simulink model "Simulink3D"  (R2013b)
settings: Solver=ode3  StartTime=0.0  StopTime=20  RelTol=1e-3
settings Model: Creator=ThiagoCordeiro  LastModifiedBy=ThiagoFelippe

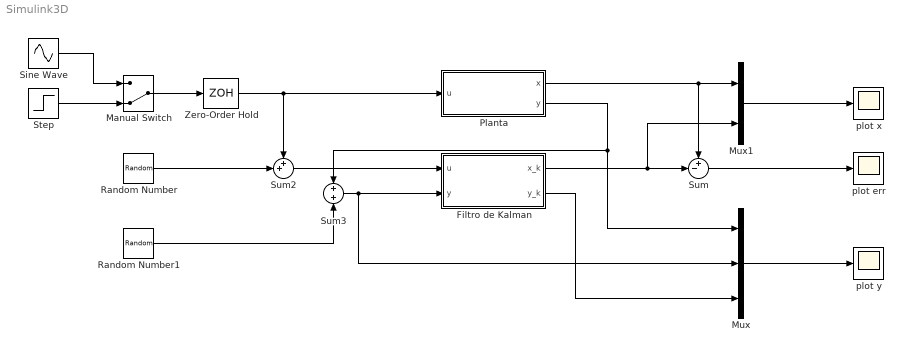
== system Simulink3D ==
  Filtro de Kalman : Subsystem
  Manual Switch : ManualSwitch  CurrentSetting=0
  Mux : Mux  Inputs=3
  Mux1 : Mux  Inputs=2
  Planta : Subsystem
  Random Number : RandomNumber  Seed=round(rand(3,1)*(2^32-1))  SampleTime=0.01
  Random Number1 : RandomNumber  Seed=round(rand(6,1)*(2^32-1))  SampleTime=0.01
  Sine Wave : Sin  Amplitude=[1 1 1]  Frequency=[1 0.5 0.25]  Phase=pi/2 * [1 1 1]  SampleTime=0
  Step : Step  Time=0  After=[2*pi/10, pi/10, pi/20]  SampleTime=0
  Sum : Sum  Inputs=+-|
  Sum2 : Sum  Inputs=++|
  Sum3 : Sum  Inputs=+|+
  Zero-Order Hold : ZeroOrderHold  SampleTime=0.01
  plot err : Scope
  plot x : Scope
  plot y : Scope
      settings: ShowLegends=on  SaveName=ScopeData2
  wires:
  Mux/1 -> plot y/1
  Zero-Order Hold/1 -> Planta/1(u), Sum2/1
  Random Number/1 -> Sum2/2
  Random Number1/1 -> Sum3/2
  Sum2/1 -> Filtro de Kalman/1(u)
  Sum3/1 -> Mux/2, Filtro de Kalman/2(y)
  Planta/2(y) -> Mux/1, Sum3/1
  Planta/1(x) -> Sum/1, Mux1/1
  Filtro de Kalman/1(x_k) -> Sum/2, Mux1/2
  Mux1/1 -> plot x/1
  Filtro de Kalman/2(y_k) -> Mux/3
  Sum/1 -> plot err/1
  Manual Switch/1 -> Zero-Order Hold/1
  Sine Wave/1 -> Manual Switch/1
  Step/1 -> Manual Switch/2

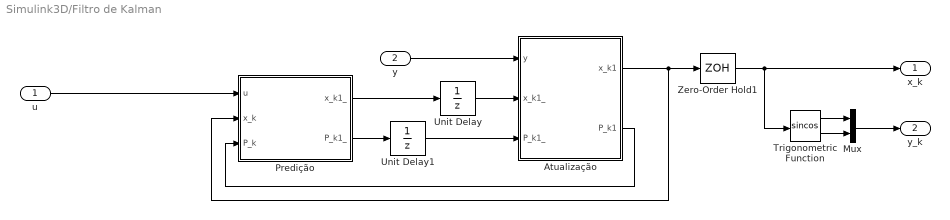
== system Simulink3D/Filtro de Kalman ==
  u : Inport
  y : Inport  Port=2
  Atualização : Subsystem
  Mux : Mux  Inputs=2
  Predição : Subsystem
  Trigonometric Function : Trigonometry  Operator=sincos
  Unit Delay : UnitDelay  InitialCondition=randn(3,1)  SampleTime=0.01
  Unit Delay1 : UnitDelay  InitialCondition=eye(3)  SampleTime=0.01
  Zero-Order Hold1 : ZeroOrderHold  SampleTime=0.01
  x_k : Outport
  y_k : Outport  Port=2
  wires:
  u/1 -> Predição/1(u)
  y/1 -> Atualização/1(y)
  Atualização/1(x_k1) -> Predição/2(x_k), Zero-Order Hold1/1
  Atualização/2(P_k1) -> Predição/3(P_k)
  Predição/2(P_k1_) -> Unit Delay1/1
  Unit Delay1/1 -> Atualização/3(P_k1_)
  Unit Delay/1 -> Atualização/2(x_k1_)
  Predição/1(x_k1_) -> Unit Delay/1
  Zero-Order Hold1/1 -> Trigonometric Function/1, x_k/1
  Mux/1 -> y_k/1
  Trigonometric Function/1 -> Mux/1
  Trigonometric Function/2 -> Mux/2

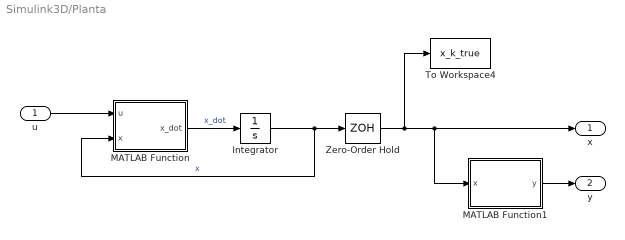
== system Simulink3D/Planta ==
  u : Inport
  Integrator : Integrator  InitialCondition=[0 0 0]
  MATLAB Function : MATLAB Function  TreatAsAtomicUnit=on
  MATLAB Function1 : MATLAB Function  TreatAsAtomicUnit=on
  To Workspace4 : ToWorkspace  VariableName=x_k_true  SampleTime=-1  SaveFormat=Timeseries
  Zero-Order Hold : ZeroOrderHold  SampleTime=0.01
  x : Outport
  y : Outport  Port=2
  wires:
  MATLAB Function/1(x_dot) -> Integrator/1  "x_dot"
  Integrator/1 -> Zero-Order Hold/1, MATLAB Function/2(x)  "x"
  u/1 -> MATLAB Function/1(u)
  MATLAB Function1/1(y) -> y/1
  Zero-Order Hold/1 -> MATLAB Function1/1(x), x/1, To Workspace4/1

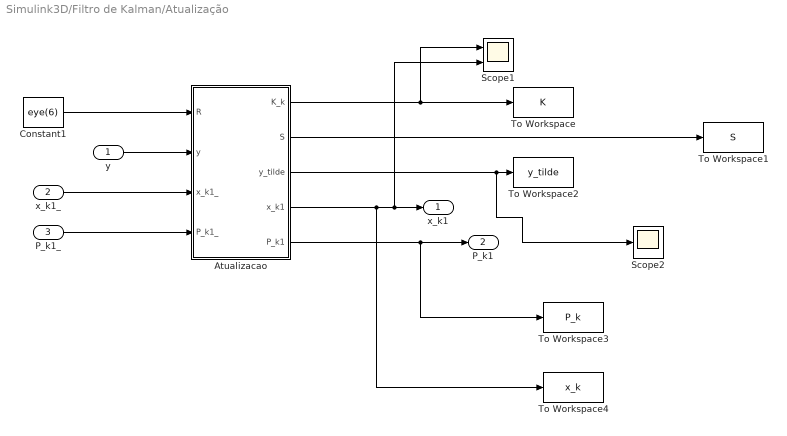
== system Simulink3D/Filtro de Kalman/Atualização ==
  y : Inport
  x_k1_ : Inport  Port=2
  P_k1_ : Inport  Port=3
  Atualizacao : MATLAB Function  TreatAsAtomicUnit=on  SystemSampleTime=0.01
  Constant1 : Constant  Value=eye(6)
  Scope1 : Scope  NumInputPorts=2
      settings: YMin=-5~-5  YMax=5~5  SaveName=ScopeData3
  Scope2 : Scope
      settings: SaveName=ScopeData5
  To Workspace : ToWorkspace  VariableName=K  SampleTime=-1  SaveFormat=Timeseries
  To Workspace1 : ToWorkspace  VariableName=S  SampleTime=-1  SaveFormat=Timeseries
  To Workspace2 : ToWorkspace  VariableName=y_tilde  SampleTime=-1  SaveFormat=Timeseries
  To Workspace3 : ToWorkspace  VariableName=P_k  SampleTime=-1  SaveFormat=Timeseries
  To Workspace4 : ToWorkspace  VariableName=x_k  SampleTime=-1  SaveFormat=Timeseries
  x_k1 : Outport
  P_k1 : Outport  Port=2
  wires:
  y/1 -> Atualizacao/2(y)
  x_k1_/1 -> Atualizacao/3(x_k1_)
  P_k1_/1 -> Atualizacao/4(P_k1_)
  Atualizacao/4(x_k1) -> To Workspace4/1, Scope1/2, x_k1/1
  Atualizacao/5(P_k1) -> To Workspace3/1, P_k1/1
  Constant1/1 -> Atualizacao/1(R)
  Atualizacao/1(K_k) -> Scope1/1, To Workspace/1
  Atualizacao/2(S) -> To Workspace1/1
  Atualizacao/3(y_tilde) -> Scope2/1, To Workspace2/1

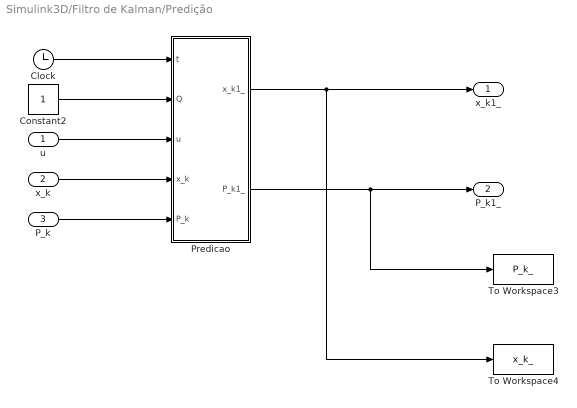
== system Simulink3D/Filtro de Kalman/Predição ==
  u : Inport
  x_k : Inport  Port=2
  P_k : Inport  Port=3
  Clock : Clock
  Constant2 : Constant
  Predicao : MATLAB Function  TreatAsAtomicUnit=on  SystemSampleTime=0.01
  To Workspace3 : ToWorkspace  VariableName=P_k_  SampleTime=-1  SaveFormat=Timeseries
  To Workspace4 : ToWorkspace  VariableName=x_k_  SampleTime=-1  SaveFormat=Timeseries
  x_k1_ : Outport
  P_k1_ : Outport  Port=2
  wires:
  u/1 -> Predicao/3(u)
  x_k/1 -> Predicao/4(x_k)
  P_k/1 -> Predicao/5(P_k)
  Constant2/1 -> Predicao/2(Q)
  Predicao/1(x_k1_) -> To Workspace4/1, x_k1_/1
  Predicao/2(P_k1_) -> To Workspace3/1, P_k1_/1
  Clock/1 -> Predicao/1(t)

== matlab function Simulink3D/Filtro de Kalman/Atualização/Atualizacao ==
  data: R input; K_k output; S output; y_tilde output; y input; x_k1_ input; P_k1_ input; x_k1 output; P_k1 output
function [K_k, S, y_tilde, x_k1, P_k1] = fcn(R, y, x_k1_, P_k1_)
%#codegen
phi = x_k1_(1);
the = x_k1_(2);
psi = x_k1_(3);

D_NED_b = DCM(phi, the, psi);

m_b = D_NED_b * [1 0 0]';
a_b = D_NED_b * [0 0 -1]';

y_hat = [m_b; a_b];

H = [ h_mag(phi, the, psi);
      h_acc(phi, the) ];

S = H * P_k1_ * H' + R;
Pxy = P_k1_ * H';
K_k  =  Pxy / S;
KH = K_k*H;
I = eye(size(KH));
I_KH = I - KH;
P_k1 = I_KH * P_k1_ * I_KH' + K_k * R * K_k';


y_tilde = y - y_hat;
x_k1 = x_k1_ + K_k * y_tilde; 

end


function D_NED_b = DCM(phi, theta, psi)

D_phi = [1 0 0;0 cos(phi) sin(phi); 0 -sin(phi) cos(phi)];
D_theta = [cos(theta) 0 -sin(theta); 0 1 0; sin(theta) 0 cos(theta)];
D_psi = [cos(psi) sin(psi) 0; -sin(psi) cos(psi) 0; 0 0 1];
D_NED_b = D_phi*D_theta*D_psi;

end

function H = h_mag(phi, the, psi)

sPs = sin(psi);
cPs = cos(psi);
sTh = sin(the);
cTh = cos(the);
sPh = sin(phi);
cPh = cos(phi);

H = [0                          -cPs*sTh        -sPs*cTh;
      cPs*sTh*cPh + sPs*sPh     cPs*cTh*sPh     -sPs*sTh*sPh - cPs*cPh;
     -cPs*sTh*sPh + sPs*cPh     cPs*cTh*cPh     -sPs*sTh*cPh + cPs*sPh];
end

function H = h_acc(phi, the)

sTh = sin(the);
cTh = cos(the);
sPh = sin(phi);
cPh = cos(phi);

H = [ 0         cTh         0;
     -cTh*cPh   sTh*sPh     0;
      cTh*sPh   sTh*cPh     0];
end

== matlab function Simulink3D/Filtro de Kalman/Predição/Predicao ==
  data: t input; Q input; u input; x_k1_ output; x_k input; P_k input; P_k1_ output
function [x_k1_,P_k1_] = fcn(t, Q, u, x_k, P_k)
%#codegen


if t >= 0
    T = 0.01;
    phi = x_k(1);
    the = x_k(2);
    psi = x_k(3);
    dp = u(1)*T;
    dq = u(2)*T;
    dr = u(3)*T;
    A = [1 tan(the)*sin(phi)    tan(the)*sin(phi);
         0 cos(phi)             -sin(phi);
         0 sin(phi)/cos(the)    cos(phi)/cos(the)];
    G = A * T; 
    x_k1_ = x_k + G*u;
    
    F_11 = 1 + tan(the) * (cos(phi)*dq - sin(phi)*dr);
    F_12 = (sec(the))^2 * (sin(phi)*dq + cos(phi)*dr);
    F_13 = 0;
    
    F_21 = -sin(phi)*dq - cos(phi)*dr;
    F_22 = 1;
    F_23 = 0;
    
    F_31 = sec(the)*(cos(phi)*dq - sin(phi)*dr);
    F_32 = sec(the)*tan(the)*(sin(phi) * dq + cos(phi)*dr);
    F_33 = 1;
    
    F = [F_11 F_12 F_13; F_21 F_22 F_23; F_31 F_32 F_33];
    
    P_k1_ = F*P_k*F' + G*Q*G';
else
    x_k1_ = x_k;
    P_k1_ = P_k;
end

== matlab function Simulink3D/Planta/MATLAB Function ==
  data: u input; x input; x_dot output
function x_dot = fcn(u,x)
%#codegen

phi = x(1);
the = x(2);
%psi = x(3);
A = [1 tan(the)*sin(phi)    tan(the)*sin(phi);
     0 cos(phi)             -sin(phi);
     0 sin(phi)/cos(the)    cos(phi)/cos(the)];
x_dot = A*u;

== matlab function Simulink3D/Planta/MATLAB Function1 ==
  data: x input; y output
function y = fcn(x)
%#codegen

D_NED_b = DCM(x(1), x(2), x(3));

m_b = D_NED_b * [1 0 0]';
a_b = D_NED_b * [0 0 -1]';

y = [m_b; a_b];

end

function D_NED_b = DCM(phi, theta, psi)

D_phi = [1 0 0;0 cos(phi) sin(phi); 0 -sin(phi) cos(phi)];
D_theta = [cos(theta) 0 -sin(theta); 0 1 0; sin(theta) 0 cos(theta)];
D_psi = [cos(psi) sin(psi) 0; -sin(psi) cos(psi) 0; 0 0 1];
D_NED_b = D_phi*D_theta*D_psi;

end
